simulink model "nonUsedBlocks"  (R2023b)
settings: Solver=VariableStepAuto  StartTime=0.0  StopTime=10.0  RelTol=1e-3
undefined symbols (not defined in the file or in its folder): A_bar, AEFF, B_E, C_bar, C_T, Cd_neg, Cd_pos, DiscIntNeverNeededParam, Gamma, H, L_gain, L_STROKE, M, m3PsToLpm, P_return_Pa, P_supply_Pa, PA_Pa, PB_Pa, RHO, Ts, V01, V02, W
(part 1 of 2)
settings Model: Creator=snr  LastModifiedBy=snr

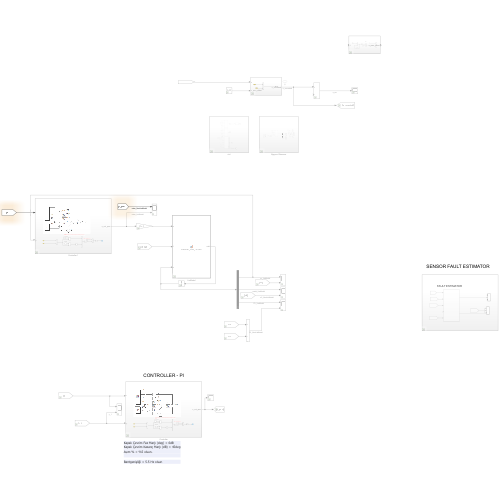
[thumbnail: Simulink's stored preview of the top-level diagram]
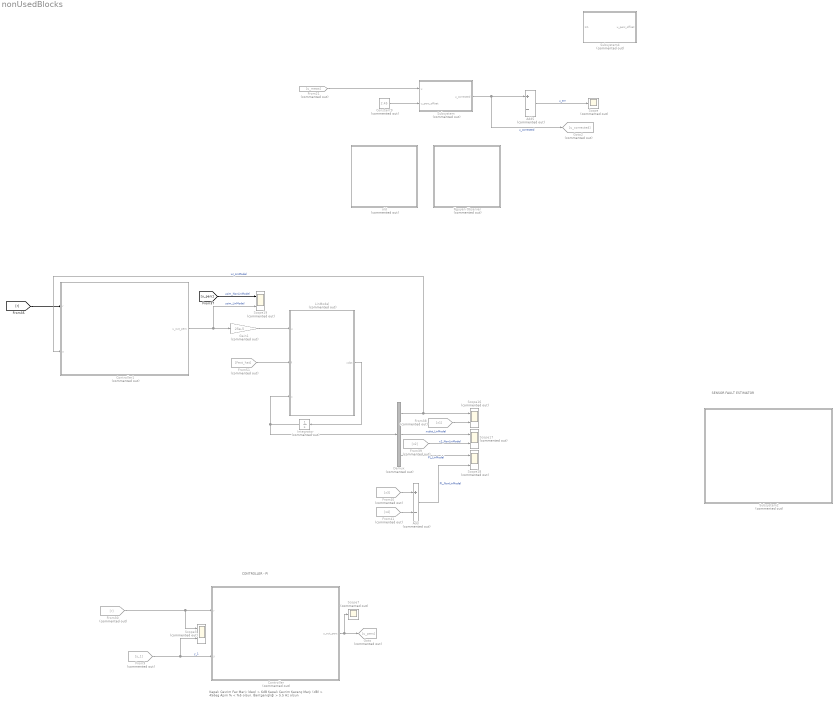
== system nonUsedBlocks ==
  note: Kapalı Çevrim Faz Marjı (deg) > 6dB
      | Kapalı Çevrim Kazanç Marjı (dB) > 45deg
      | Aşım % < %5 olsun.
      |
      | Bantgenişliği > 5.5 Hz olsun
  note: CONTROLLER - PI
  note: SENSOR FAULT ESTIMATOR
  Add : Sum  Commented=on  Inputs=+-
  Add5 : Sum  Commented=on  Inputs=+-
  Constant9 : Constant  Commented=on  Value=2.45
  Controller : Subsystem  Commented=on
  Controller1 : Subsystem  Commented=on
  Demux : Demux  Commented=on  Outputs=3
  From21 : From  Commented=on  GotoTag=u_meas
  From30 : From  Commented=on  GotoTag=r
  From38 : From  Commented=on  GotoTag=x1
  From39 : From  Commented=on  GotoTag=x2
  From40 : From  Commented=on  GotoTag=x3
  From41 : From  Commented=on  GotoTag=x4
  From51 : From  Commented=on  GotoTag=Fext_hat
  From9 : From  Commented=on  GotoTag=y_1
  Gain1 : Gain  Commented=on  Gain=25e-5
  Goto : Goto  Commented=on  GotoTag=u_perc
  Goto2 : Goto  Commented=on  GotoTag=u_corrected
  Integrator : Integrator  Commented=on  InitialCondition=[0;0;0]
  LinModel : MATLAB Function  Commented=on  TreatAsAtomicUnit=on
  Nguyen Observer : Subsystem  Commented=on
  Scope : Scope  Commented=on
  Scope{3,16..19} (5 alike) : Scope  Commented=on  NumInputPorts=2
  Scope7 : Scope  Commented=on
  Subsystem : Subsystem  Commented=on
  Subsystem2 : Subsystem  Commented=on
  Subsystem4 : Subsystem  Commented=on
  old : Subsystem  Commented=on
  wires:
  Controller1/1(u_out_perc) -> Scope19/2, Gain1/1  "usim_LinModel"
  [r] -> Controller1/1(r)
  Integrator/1 -> LinModel/3(x), Demux/1
  Demux/2 -> Scope17/1  "xcdot_LinModel"
  LinModel/1(xdot) -> Integrator/1
  From40/1 -> Add/1
  From41/1 -> Add/2
  Demux/1 -> Controller1/2(y), Scope16/1  "xc_LinModel"
  Add/1 -> Scope18/2  "PL_NonLinModel"
  Gain1/1 -> LinModel/1(u)
  From51/1 -> LinModel/2(f)
  From38/1 -> Scope16/2
  [u_perc] -> Scope19/1  "usim_NonLinModel"
  From30/1 -> Scope3/1, Controller/1(r)
  Constant9/1 -> Subsystem/2(u_perc_offset)
  Demux/3 -> Scope18/1  "PL_LinModel"
  Subsystem/1(u_corrected) -> Goto2/1, Add5/1  "u_corrected"
  Controller/1(u_out_perc) -> Scope7/1, Goto/1
  From39/1 -> Scope17/2  "x2_NonLinModel"
  Add5/1 -> Scope/1  "u_err"
  From21/1 -> Subsystem/1(u)
  From9/1 -> Scope3/2, Controller/2(y)  "y_1"

== system nonUsedBlocks/Controller ==
  note: Kontrolcü kazançları Kp : 5 - Ki :40 test düzeneğinde, Sim ortamında uygunluk için böyle ayarladım
  note: Offset - Yapmaya İhtiyaç yok
  note: Integral Gain
  note: Proportional Gain
  r : Inport  OutDataTypeStr=double
  y : Inport  Port=2  OutDataTypeStr=double
  Add : Sum
  Add1 : Sum  Inputs=+-
  Add3 : Sum
  Constant : Constant  Value=45
  Constant1 : Constant  Value=5
  Constant2 : Constant  Value=0  OutDataTypeStr=double
  Gain1 : Gain  Gain=1000
  Integrator : Integrator
  Product : Product
  Product1 : Product
  Saturation : Saturate  UpperLimit=100  LowerLimit=-100
  u_out_perc : Outport  OutDataTypeStr=double
  wires:
  Constant/1 -> Product/1
  Constant1/1 -> Product1/1
  Add1/1 -> Product1/2, Product/2  "e"
  Product/1 -> Integrator/1
  Integrator/1 -> Add/2
  r/1 -> Add1/1  "r"
  Add/1 -> Gain1/1
  y/1 -> Add1/2
  Add3/1 -> Saturation/1
  Gain1/1 -> Add3/2
  Saturation/1 -> u_out_perc/1
  Product1/1 -> Add/1
  Constant2/1 -> Add3/1

== system nonUsedBlocks/Controller1 ==
  note: Proportional Gain
  note: Integral Gain
  note: Offset - Yapmaya İhtiyaç yok
  note: Kontrolcü kazançları Kp : 5 - Ki :40 test düzeneğinde, Sim ortamında uygunluk için böyle ayarladım
  r : Inport  OutDataTypeStr=double
  y : Inport  Port=2  OutDataTypeStr=double
  Add : Sum
  Add1 : Sum  Inputs=+-
  Add3 : Sum
  Constant : Constant  Value=45
  Constant1 : Constant  Value=5
  Constant2 : Constant  Value=0  OutDataTypeStr=double
  Gain1 : Gain  Gain=1000
  Integrator : Integrator
  Product : Product
  Product1 : Product
  Saturation : Saturate  UpperLimit=100  LowerLimit=-100
  u_out_perc : Outport  OutDataTypeStr=double
  wires:
  Constant2/1 -> Add3/1
  Product1/1 -> Add/1
  Saturation/1 -> u_out_perc/1
  Gain1/1 -> Add3/2
  Add3/1 -> Saturation/1
  y/1 -> Add1/2
  Add/1 -> Gain1/1
  r/1 -> Add1/1  "r"
  Integrator/1 -> Add/2
  Product/1 -> Integrator/1
  Add1/1 -> Product/2, Product1/2  "e"
  Constant1/1 -> Product1/1
  Constant/1 -> Product/1

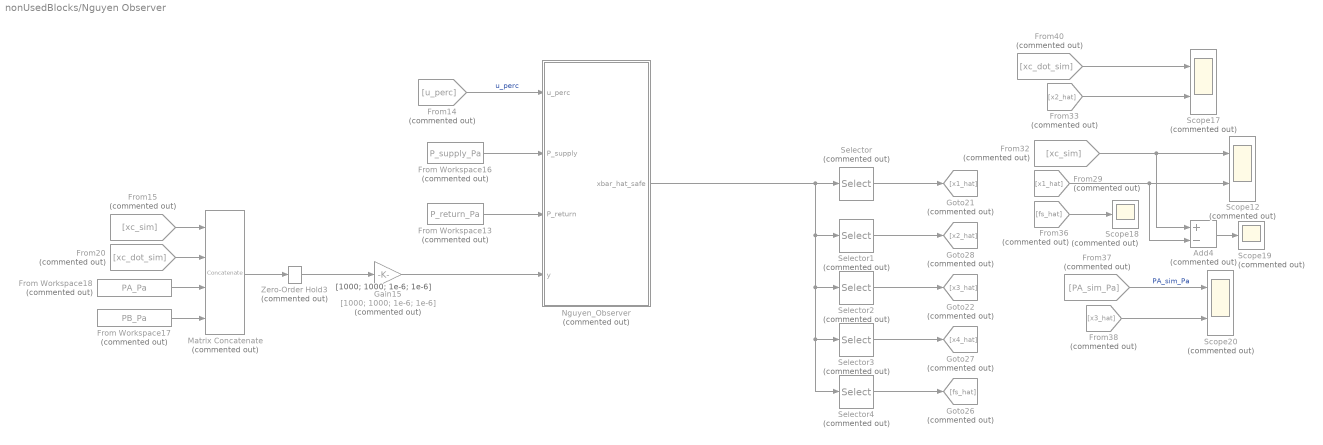
== system nonUsedBlocks/Nguyen Observer ==
  note: [1000; 1000; 1e-6; 1e-6]
  Add4 : Sum  Commented=on  Inputs=+-
  From Workspace13 : FromWorkspace  Commented=on  VariableName=P_return_Pa
  From Workspace16 : FromWorkspace  Commented=on  VariableName=P_supply_Pa
  From Workspace17 : FromWorkspace  Commented=on  VariableName=PB_Pa
  From Workspace18 : FromWorkspace  Commented=on  VariableName=PA_Pa
  From14 : From  Commented=on  GotoTag=u_perc
  From15 : From  Commented=on  GotoTag=xc_sim
  From20 : From  Commented=on  GotoTag=xc_dot_sim
  From29 : From  Commented=on  GotoTag=x1_hat
  From32 : From  Commented=on  GotoTag=xc_sim
  From33 : From  Commented=on  GotoTag=x2_hat
  From36 : From  Commented=on  GotoTag=fs_hat
  From37 : From  Commented=on  GotoTag=PA_sim_Pa
  From38 : From  Commented=on  GotoTag=x3_hat
  From40 : From  Commented=on  GotoTag=xc_dot_sim
  Gain15 : Gain  Commented=on  Gain=[1000; 1000; 1e-6; 1e-6]
  Goto21 : Goto  Commented=on  GotoTag=x1_hat
  Goto22 : Goto  Commented=on  GotoTag=x3_hat
  Goto26 : Goto  Commented=on  GotoTag=fs_hat
  Goto27 : Goto  Commented=on  GotoTag=x4_hat
  Goto28 : Goto  Commented=on  GotoTag=x2_hat
  Matrix Concatenate : Concatenate  Commented=on  NumInputs=4  Mode=Multidimensional array
  Nguyen_Observer : Subsystem  Commented=on
  Scope12 : Scope  Commented=on  NumInputPorts=2
  Scope17 : Scope  Commented=on  NumInputPorts=2
  Scope18 : Scope  Commented=on
  Scope19 : Scope  Commented=on
  Scope20 : Scope  Commented=on  NumInputPorts=2
  Selector : Selector  Commented=on  InputPortWidth=5  IndexOptions=Index vector (dialog)  Indices=1  OutputSizes=1
  Selector1 : Selector  Commented=on  InputPortWidth=5  IndexOptions=Index vector (dialog)  Indices=2  OutputSizes=1
  Selector2 : Selector  Commented=on  InputPortWidth=5  IndexOptions=Index vector (dialog)  Indices=3  OutputSizes=1
  Selector3 : Selector  Commented=on  InputPortWidth=5  IndexOptions=Index vector (dialog)  Indices=4  OutputSizes=1
  Selector4 : Selector  Commented=on  InputPortWidth=5  IndexOptions=Index vector (dialog)  Indices=5  OutputSizes=1
  Zero-Order Hold3 : ZeroOrderHold  Commented=on  SampleTime=Ts
  wires:
  From Workspace13/1 -> Nguyen_Observer/3(P_return)
  Add4/1 -> Scope19/1
  From Workspace17/1 -> Matrix Concatenate/4
  Selector4/1 -> Goto26/1
  From14/1 -> Nguyen_Observer/1(u_perc)  "u_perc"
  Selector2/1 -> Goto22/1
  Matrix Concatenate/1 -> Zero-Order Hold3/1
  From38/1 -> Scope20/2
  From Workspace16/1 -> Nguyen_Observer/2(P_supply)
  From32/1 -> Add4/1, Scope12/1
  Zero-Order Hold3/1 -> Gain15/1
  From36/1 -> Scope18/1
  From40/1 -> Scope17/1
  Gain15/1 -> Nguyen_Observer/4(y)
  From20/1 -> Matrix Concatenate/2
  From15/1 -> Matrix Concatenate/1
  Selector/1 -> Goto21/1
  Selector3/1 -> Goto27/1
  From37/1 -> Scope20/1  "PA_sim_Pa"
  Selector1/1 -> Goto28/1
  From Workspace18/1 -> Matrix Concatenate/3
  Nguyen_Observer/1(xbar_hat_safe) -> Selector4/1, Selector3/1, Selector2/1, Selector1/1, Selector/1
  From33/1 -> Scope17/2
  From29/1 -> Add4/2, Scope12/2

== system nonUsedBlocks/Subsystem ==
  u : Inport  OutDataTypeStr=double
  u_perc_offset : Inport  Port=2  OutDataTypeStr=double
  Add : Sum  Inputs=+-
  u_corrected : Outport
  wires:
  u/1 -> Add/1
  u_perc_offset/1 -> Add/2
  Add/1 -> u_corrected/1

== system nonUsedBlocks/Subsystem2 ==
  note: FAULT ESTIMATOR
  From14 : From  Commented=on  GotoTag=u_perc
  From15 : From  Commented=on  GotoTag=PA_sim_Pa
  From20 : From  Commented=on  GotoTag=PB_sim_Pa
  From29 : From  Commented=on  GotoTag=fs_real
  From33 : From  Commented=on  GotoTag=xc_dot_sim
  Scope12 : Scope  Commented=on  NumInputPorts=3
  Scope17 : Scope  Commented=on  NumInputPorts=3
  Subsystem3 : Subsystem  Commented=on
  wires:
  Subsystem3/2(Out1) -> Scope17/1
  From20/1 -> Subsystem3/3(PB_Pa)  "PB_sim_Pa"
  From29/1 -> Subsystem3/5(fs_real)
  From14/1 -> Subsystem3/1(u_real)  "u_perc"
  From33/1 -> Scope17/2
  From15/1 -> Subsystem3/2(PA_Pa)
  Subsystem3/1(x_bar) -> Scope12/2  "x_bar"

== system nonUsedBlocks/Subsystem4 ==
  In1 : Inport
  Add : Sum
  Constant : Constant
  Constant1 : Constant  Value=100
  Relational Operator : RelationalOperator  OutDataTypeStr=boolean  RndMeth=Simplest  InputSameDT=off
  Saturation : Saturate  UpperLimit=100  LowerLimit=0
  Switch : Switch  Criteria=u2 ~= 0  SaturateOnIntegerOverflow=off  InputSameDT=off
  Unit Delay : UnitDelay  SampleTime=-1  HasFrameUpgradeWarning=on
  u_perc_offset : Outport
  wires:
  Constant/1 -> Add/1
  Add/1 -> Unit Delay/1, Saturation/1
  Unit Delay/1 -> Add/2
  Saturation/1 -> Relational Operator/1
  Constant1/1 -> Relational Operator/2
  Relational Operator/1 -> Switch/2
  In1/1 -> Switch/1

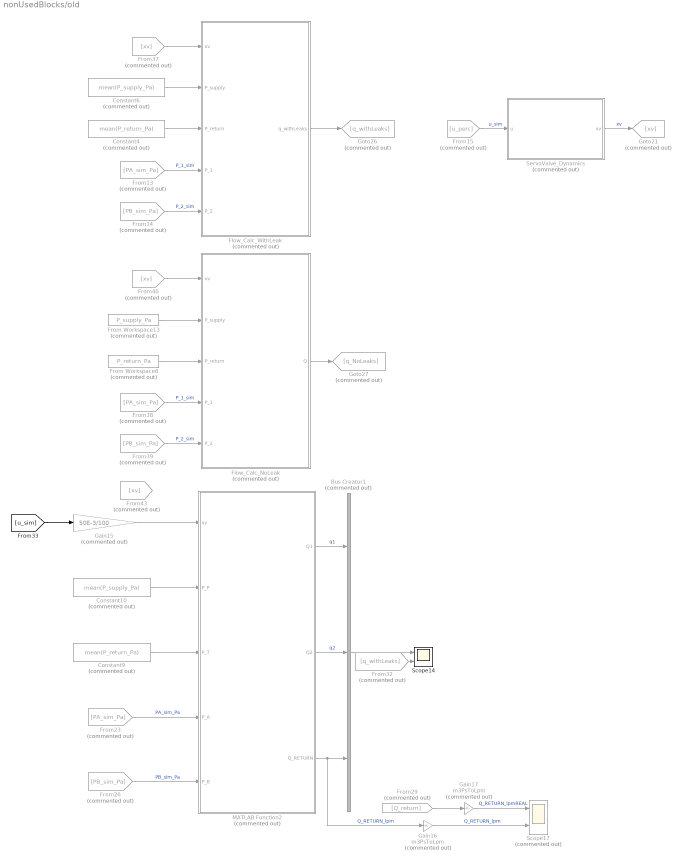
== system nonUsedBlocks/old ==
  Bus Creator1 : BusCreator  Commented=on  Inputs=3
  Constant10 : Constant  Commented=on  Value=mean(P_supply_Pa)
  Constant4 : Constant  Commented=on  Value=mean(P_return_Pa)
  Constant6 : Constant  Commented=on  Value=mean(P_supply_Pa)
  Constant9 : Constant  Commented=on  Value=mean(P_return_Pa)
  Flow_Calc_NoLeak : Subsystem  Commented=on
  Flow_Calc_WithLeak : Subsystem  Commented=on
  From Workspace13 : FromWorkspace  Commented=on  VariableName=P_supply_Pa
  From Workspace8 : FromWorkspace  Commented=on  VariableName=P_return_Pa
  From13 : From  Commented=on  GotoTag=PA_sim_Pa
  From14 : From  Commented=on  GotoTag=PB_sim_Pa
  From15 : From  Commented=on  GotoTag=u_perc
  From23 : From  Commented=on  GotoTag=PA_sim_Pa
  From26 : From  Commented=on  GotoTag=PB_sim_Pa
  From29 : From  Commented=on  GotoTag=Q_return
  From32 : From  Commented=on  GotoTag=q_withLeaks
  From37 : From  Commented=on  GotoTag=xv
  From38 : From  Commented=on  GotoTag=PA_sim_Pa
  From39 : From  Commented=on  GotoTag=PB_sim_Pa
  From40 : From  Commented=on  GotoTag=xv
  From43 : From  Commented=on  GotoTag=xv
  Gain15 : Gain  Commented=on  Gain=50E-3/100
  Gain16 : Gain  Commented=on  Gain=m3PsToLpm
  Gain17 : Gain  Commented=on  Gain=m3PsToLpm
  Goto21 : Goto  Commented=on  GotoTag=xv
  Goto26 : Goto  Commented=on  GotoTag=q_withLeaks
  Goto27 : Goto  Commented=on  GotoTag=q_NoLeaks
  MATLAB Function2 : MATLAB Function  Commented=on  TreatAsAtomicUnit=on
  Scope14 : Scope  NumInputPorts=2
  Scope17 : Scope  Commented=on  NumInputPorts=2
  ServoValve_Dynamics : Subsystem  Commented=on
  wires:
  Constant9/1 -> MATLAB Function2/3(P_T)
  From32/1 -> Scope14/2
  Constant4/1 -> Flow_Calc_WithLeak/3(P_return)
  From26/1 -> MATLAB Function2/5(P_B)  "PB_sim_Pa"
  From Workspace13/1 -> Flow_Calc_NoLeak/2(P_supply)
  From29/1 -> Gain17/1
  Gain15/1 -> MATLAB Function2/1(xv)
  Bus Creator1/1 -> Scope14/1
  From37/1 -> Flow_Calc_WithLeak/1(xv)
  Constant10/1 -> MATLAB Function2/2(P_P)
  From Workspace8/1 -> Flow_Calc_NoLeak/3(P_return)
  MATLAB Function2/3(Q_RETURN) -> Gain16/1, Bus Creator1/3  "Q_RETURN_lpm"
  From23/1 -> MATLAB Function2/4(P_A)  "PA_sim_Pa"
  Gain16/1 -> Scope17/2  "Q_RETURN_lpm"
  MATLAB Function2/1(Q1) -> Bus Creator1/1  "q1"
  MATLAB Function2/2(Q2) -> Bus Creator1/2  "q2"
  From14/1 -> Flow_Calc_WithLeak/5(P_2)  "P_2_sim"
  From39/1 -> Flow_Calc_NoLeak/5(P_2)  "P_2_sim"
  Flow_Calc_NoLeak/1(Q) -> Goto27/1
  Flow_Calc_WithLeak/1(q_withLeaks) -> Goto26/1
  From40/1 -> Flow_Calc_NoLeak/1(xv)
  [u_sim] -> Gain15/1
  Constant6/1 -> Flow_Calc_WithLeak/2(P_supply)
  From38/1 -> Flow_Calc_NoLeak/4(P_1)  "P_1_sim"
  From13/1 -> Flow_Calc_WithLeak/4(P_1)  "P_1_sim"
  Gain17/1 -> Scope17/1  "Q_RETURN_lpmREAL"
  ServoValve_Dynamics/1(xv) -> Goto21/1  "xv"
  From15/1 -> ServoValve_Dynamics/1(u)  "u_sim"

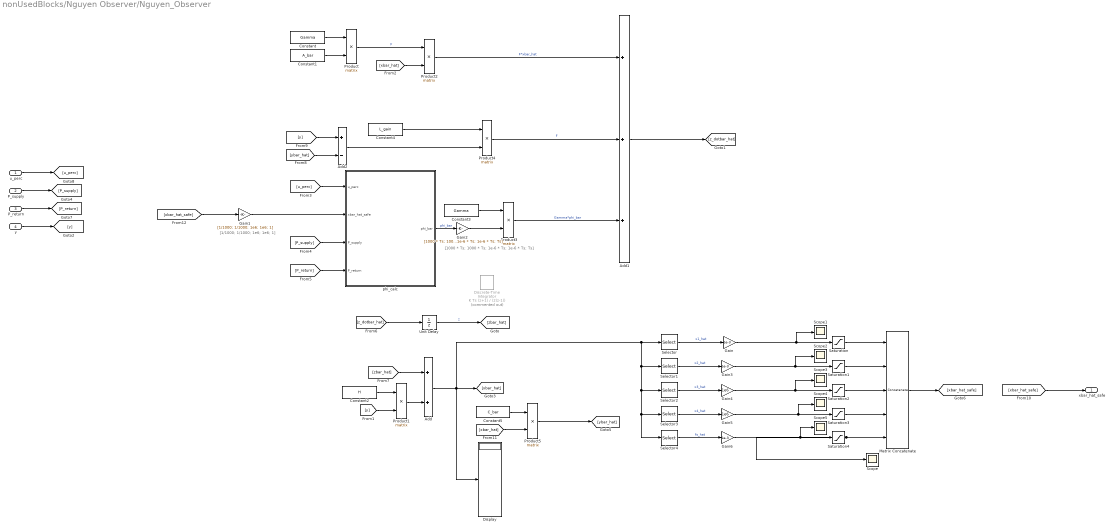
== system nonUsedBlocks/Nguyen Observer/Nguyen_Observer ==
  note: [1000 * Ts; 1000 * Ts; 1e-6 * Ts; 1e-6 * Ts; Ts]
  note: [1/1000; 1/1000; 1e6; 1e6; 1]
  u_perc : Inport  PortDimensions=[1,1]
  P_supply : Inport  Port=2  OutDataTypeStr=double
  P_return : Inport  Port=3  OutDataTypeStr=double
  y : Inport  Port=4  PortDimensions=[4,1]
  Add : Sum
  Add1 : Sum  Inputs=+++
  Add2 : Sum  Inputs=+-
  Constant : Constant  Value=Gamma
  Constant1 : Constant  Value=A_bar
  Constant2 : Constant  Value=H
  Constant3 : Constant  Value=Gamma
  Constant4 : Constant  Value=L_gain
  Constant5 : Constant  Value=C_bar
  Discrete-Time Integrator : DiscreteIntegrator  Commented=on  IntegratorMethod=Integration: Trapezoidal  InitialCondition=[0,0,PA_Pa.Data(1)*1e-6,PB_Pa.Data(1)*1e-6,0]'  SampleTime=-1  ICPrevOutput=DiscIntNeverNeededParam  ICPrevScaledInput=DiscIntNeverNeededParam
  Display : Display
  Gain : Gain  Gain=1e-3
  Gain1 : Gain  Gain=[1/1000; 1/1000; 1e6; 1e6; 1]
  Gain2 : Gain  Gain=[1000 * Ts; 1000 * Ts; 1e-6 * Ts; 1e-6 * Ts; Ts]
  Gain3 : Gain  Gain=1e-3
  Gain4 : Gain  Gain=1e6
  Gain5 : Gain  Gain=1e6
  Gain6 : Gain  Gain=1e-3
  Matrix Concatenate : Concatenate  NumInputs=5  Mode=Multidimensional array
  Product{,1..5} (6 alike) : Product  Multiplication=Matrix(*)
  Saturation : Saturate  UpperLimit=L_STROKE  LowerLimit=-L_STROKE
  Saturation1 : Saturate  UpperLimit=2  LowerLimit=-2
  Saturation2 : Saturate  UpperLimit=200e5  LowerLimit=4e5
  Saturation3 : Saturate  UpperLimit=200e5  LowerLimit=4e5
  Saturation4 : Saturate  UpperLimit=L_STROKE  LowerLimit=-L_STROKE
  Scope{,1..5} (6 alike) : Scope
  Selector : Selector  InputPortWidth=5  IndexOptions=Index vector (dialog)  Indices=1  OutputSizes=1
  Selector1 : Selector  InputPortWidth=5  IndexOptions=Index vector (dialog)  Indices=2  OutputSizes=1
  Selector2 : Selector  InputPortWidth=5  IndexOptions=Index vector (dialog)  Indices=3  OutputSizes=1
  Selector3 : Selector  InputPortWidth=5  IndexOptions=Index vector (dialog)  Indices=4  OutputSizes=1
  Selector4 : Selector  InputPortWidth=5  IndexOptions=Index vector (dialog)  Indices=5  OutputSizes=1
  Unit Delay : UnitDelay  InitialCondition=[0,0,PA_Pa.Data(1)*1e-6,PB_Pa.Data(1)*1e-6,0]'  SampleTime=Ts  HasFrameUpgradeWarning=on
  phi_calc : Subsystem
  xbar_hat_safe : Outport
  wires:
  [y] -> Add2/1
  Product3/1 -> Add1/3  "Gamma*phi_bar"
  [u_perc] -> phi_calc/1(u_perc)
  Add2/1 -> Product4/2
  u_perc/1 -> [u_perc]
  Constant3/1 -> Product3/1
  Unit Delay/1 -> [zbar_hat]  "z"
  [ybar_hat] -> Add2/2
  Constant2/1 -> Product1/1
  Product/1 -> Product2/1  "F"
  [P_return] -> phi_calc/4(P_return)
  Constant1/1 -> Product/2
  Product2/1 -> Add1/1  "F*xbar_hat"
  Constant/1 -> Product/1
  [xbar_hat] -> Product2/2
  P_return/1 -> [P_return]
  [y] -> Product1/2
  [zbar_hat] -> Add/1
  y/1 -> [y]
  Add1/1 -> [z_dotbar_hat]
  Product4/1 -> Add1/2  "F"
  Product1/1 -> Add/2
  P_supply/1 -> [P_supply]
  phi_calc/1(phi_bar) -> Gain2/1  "phi_bar"
  [P_supply] -> phi_calc/3(P_supply)
  [z_dotbar_hat] -> Unit Delay/1
  [xbar_hat_safe] -> xbar_hat_safe/1
  Constant5/1 -> Product5/1
  [xbar_hat] -> Product5/2
  Product5/1 -> [ybar_hat]
  Selector3/1 -> Gain5/1  "x4_hat"
  Selector2/1 -> Gain4/1  "x3_hat"
  Selector1/1 -> Gain3/1  "x2_hat"
  Saturation/1 -> Matrix Concatenate/1
  Saturation1/1 -> Matrix Concatenate/2
  Saturation2/1 -> Matrix Concatenate/3
  Saturation3/1 -> Matrix Concatenate/4
  Saturation4/1 -> Scope/1, Matrix Concatenate/5
  Matrix Concatenate/1 -> [xbar_hat_safe]
  Selector4/1 -> Gain6/1  "fs_hat"
  Selector/1 -> Gain/1  "x1_hat"
  Constant4/1 -> Product4/1
  Add/1 -> Selector3/1, Selector4/1, Selector2/1, Selector1/1, Selector/1, [xbar_hat], Display/1
  [xbar_hat_safe] -> Gain1/1
  Gain1/1 -> phi_calc/2(xbar_hat_safe)
  Gain2/1 -> Product3/2
  Gain/1 -> Scope1/1, Saturation/1
  Gain3/1 -> Scope2/1, Saturation1/1
  Gain4/1 -> Saturation2/1, Scope3/1
  Gain5/1 -> Saturation3/1, Scope4/1
  Gain6/1 -> Scope5/1, Saturation4/1

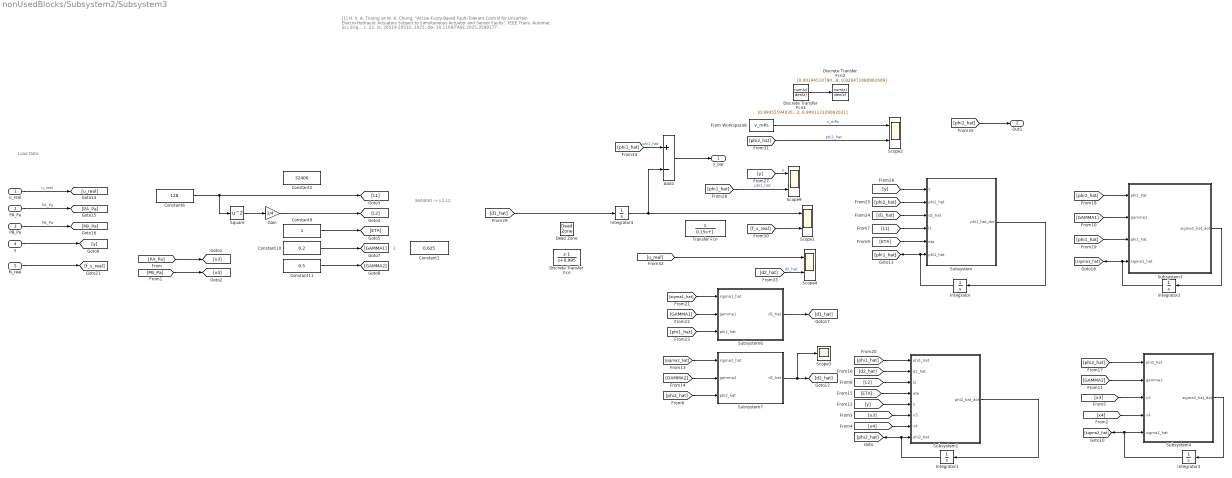
== system nonUsedBlocks/Subsystem2/Subsystem3 ==
  note: [1]
      | H. V. A. Truong ve W. K. Chung, “Active Fuzzy-Based Fault-Tolerant Control for Uncertain Electro-Hydraulic Actuators Subject to Simultaneous Actuator and Sensor Faults”, IEEE Trans. Automat. Sci. Eng. , c. 22, ss. 20519-20532, 2025, doi: 10.1109/TASE.2025.3599177 .
  note: 2
  note: 360/850 -> L1,L2
  note: Load Data
  u_real : Inport
  PA_Pa : Inport  Port=2
  PB_Pa : Inport  Port=3
  y : Inport  Port=4
  fs_real : Inport  Port=5
  Add1 : Sum  Inputs=+-
  Constant1 : Constant  Value=0.625
  Constant10 : Constant  Value=0.2
  Constant11 : Constant  Value=0.5
  Constant2 : Constant  Value=32400
  Constant6 : Constant  Value=128
  Constant9 : Constant
  Dead Zone : DeadZone  LowerValue=-0.01  UpperValue=0.01
  Discrete Transfer Fcn : DiscreteTransferFcn  Numerator=[1 -1]  Denominator=[1 0.995]
  Discrete Transfer Fcn1 : DiscreteTransferFcn  Numerator=[0.999555940307616, -1.999111880615232, 0.999555940307616]  Denominator=[1.000000000000000, -1.999111432168433, 0.999112329062031]
  Discrete Transfer Fcn2 : DiscreteTransferFcn  Numerator=[0.001945107908955, 0.003890215817911, 0.001945107908955]  Denominator=[1.000000000000000, -1.812690649346788, 0.820471080982609]
  From Workspace6 : FromWorkspace  VariableName=v_mPs
  Gain : Gain  Gain=1/4
  Integrator{,1..4} (5 alike) : Integrator
  Scope{1..2,4,9} (4 alike) : Scope  NumInputPorts=2
  Scope3 : Scope
  Square : Math  Operator=square
  Subsystem : Subsystem
  Subsystem1 : Subsystem
  Subsystem3 : Subsystem
  Subsystem4 : Subsystem
  Subsystem6 : Subsystem
  Subsystem7 : Subsystem
  Transfer Fcn : TransferFcn  Denominator=[0.15 1]
  x_bar : Outport
  Out1 : Outport  Port=2
  wires:
  [u_real] -> Scope4/1
  Subsystem4/1(sigma2_hat_dot) -> Integrator3/1
  Constant6/1 -> Square/1, [L1]
  [y] -> Subsystem/1(y)
  Constant9/1 -> [ETA]
  [GAMMA2] -> Subsystem7/2(gamma2)
  [GAMMA1] -> Subsystem3/2(gamma1)
  Subsystem/1(phi1_hat_dot) -> Integrator/1
  Gain/1 -> [L2]
  [GAMMA1] -> Subsystem6/2(gamma1)
  [y] -> Subsystem1/5(y)
  Constant10/1 -> [GAMMA1]
  y/1 -> [y]
  [GAMMA2] -> Subsystem4/2(gamma2)
  Subsystem7/1(d2_hat) -> Scope3/1, [d2_hat]
  [L2] -> Subsystem1/3(l2)
  Subsystem6/1(d1_hat) -> [d1_hat]
  [phi1_hat] -> Subsystem3/3(phi1_hat)
  [ETA] -> Subsystem/5(eta)
  [phi1_hat] -> Scope9/2  "phi1_hat"
  Integrator/1 -> [phi1_hat], Subsystem/6(phi1_hat)
  [d2_hat] -> Subsystem1/2(d2_hat)
  Constant11/1 -> [GAMMA2]
  [d2_hat] -> Scope4/2  "d2_hat"
  [phi2_hat] -> Subsystem7/3(phi2_hat)
  [y] -> Scope9/1  "y"
  [phi2_hat] -> Subsystem4/1(phi2_hat)
  [sigma1_hat] -> Subsystem6/1(sigma1_hat)
  [L1] -> Subsystem/4(l1)
  Integrator2/1 -> [sigma1_hat], Subsystem3/4(sigma1_hat)
  [PA_Pa] -> [x3]
  [x3] -> Subsystem1/6(x3)
  PB_Pa/1 -> [PB_Pa]  "PB_Pa"
  u_real/1 -> [u_real]  "u_real"
  Subsystem3/1(sigma1_hat_dot) -> Integrator2/1
  [ETA] -> Subsystem1/4(eta)
  [phi1_hat] -> Subsystem6/3(phi1_hat)
  Integrator3/1 -> Subsystem4/5(sigma2_hat), [sigma2_hat]
  [sigma2_hat] -> Subsystem7/1(sigma2_hat)
  [x3] -> Subsystem4/3(x3)
  [x4] -> Subsystem4/4(x4)
  [d1_hat] -> Subsystem/3(d1_hat)
  From Workspace6/1 -> Scope2/1  "v_mPs"
  [phi1_hat] -> Subsystem1/1(phi1_hat)
  [phi2_hat] -> Subsystem/2(phi2_hat)
  [phi2_hat] -> Subsystem3/1(phi2_hat)
  [x4] -> Subsystem1/7(x4)
  PA_Pa/1 -> [PA_Pa]  "PA_Pa"
  [PB_Pa] -> [x4]
  [phi1_hat] -> Add1/1  "phi1_hat"
  Add1/1 -> x_bar/1
  fs_real/1 -> [f_s_real]
  [phi2_hat] -> Out1/1
  Subsystem1/1(phi2_hat_dot) -> Integrator1/1
  Integrator1/1 -> Subsystem1/8(phi2_hat), [phi2_hat]
  Square/1 -> Gain/1
  [d1_hat] -> Integrator4/1
  Integrator4/1 -> Scope1/1, Add1/2
  [f_s_real] -> Scope1/2
  Discrete Transfer Fcn1/1 -> Discrete Transfer Fcn2/1
  [phi2_hat] -> Scope2/2  "phi2_hat"

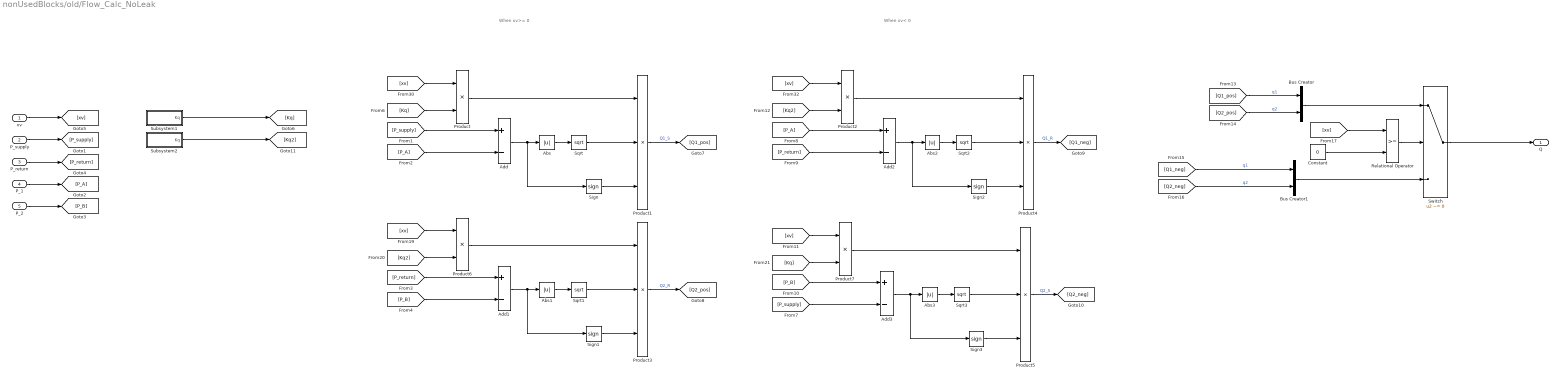
== system nonUsedBlocks/old/Flow_Calc_NoLeak ==
  note: When xv< 0
  note: When xv>= 0
  xv : Inport  OutDataTypeStr=double
  P_supply : Inport  Port=2  OutDataTypeStr=double
  P_return : Inport  Port=3  OutDataTypeStr=double
  P_1 : Inport  Port=4  OutDataTypeStr=double
  P_2 : Inport  Port=5  OutDataTypeStr=double
  Abs{,1..3} (4 alike) : Abs  SaturateOnIntegerOverflow=off
  Add{,1..3} (4 alike) : Sum  Inputs=+-
  Bus Creator : BusCreator  Inputs=2
  Bus Creator1 : BusCreator  Inputs=2
  Constant : Constant  Value=0  OutDataTypeStr=double
  Product{,2,6..7} (4 alike) : Product
  Product{1,3..5} (4 alike) : Product  Inputs=3
  Relational Operator : RelationalOperator  OutDataTypeStr=boolean  RndMeth=Simplest  InputSameDT=off
  Sign{,1..3} (4 alike) : Signum
  Sqrt{,1..3} (4 alike) : Sqrt
  Subsystem1 : Subsystem
  Subsystem2 : Subsystem
  Switch : Switch  Criteria=u2 ~= 0  SaturateOnIntegerOverflow=off  InputSameDT=off
  Q : Outport  OutDataTypeStr=double
  wires:
  Subsystem2/1(Kq) -> [Kq2]
  Subsystem1/1(Kq) -> [Kq]
  Product5/1 -> [Q2_neg]  "Q2_S"
  Product4/1 -> [Q1_neg]  "Q1_R"
  Product3/1 -> [Q2_pos]  "Q2_R"
  Product1/1 -> [Q1_pos]  "Q1_S"
  Switch/1 -> Q/1
  [xv] -> Product/1
  [Q1_neg] -> Bus Creator1/1  "q1"
  [Q2_pos] -> Bus Creator/2  "q2"
  Product7/1 -> Product5/1
  [xv] -> Product7/1
  [Kq] -> Product7/2
  Product6/1 -> Product3/1
  [Kq2] -> Product6/2
  [xv] -> Product6/1
  Bus Creator1/1 -> Switch/3
  Bus Creator/1 -> Switch/1
  Relational Operator/1 -> Switch/2
  Constant/1 -> Relational Operator/2
  [xv] -> Relational Operator/1
  [Q2_neg] -> Bus Creator1/2  "q2"
  [Q1_pos] -> Bus Creator/1  "q1"
  [P_supply] -> Add3/2
  [P_B] -> Add3/1
  [P_return] -> Add2/2
  [P_A] -> Add2/1
  Product2/1 -> Product4/1
  Sqrt2/1 -> Product4/2
  Abs2/1 -> Sqrt2/1
  Add2/1 -> Abs2/1, Sign2/1
  Sign2/1 -> Product4/3
  Sign3/1 -> Product5/3
  Add3/1 -> Sign3/1, Abs3/1
  Abs3/1 -> Sqrt3/1
  Sqrt3/1 -> Product5/2
  [Kq2] -> Product2/2
  [xv] -> Product2/1
  xv/1 -> [xv]
  P_return/1 -> [P_return]
  P_2/1 -> [P_B]
  P_1/1 -> [P_A]
  P_supply/1 -> [P_supply]
  [P_B] -> Add1/2
  [P_return] -> Add1/1
  [Kq] -> Product/2
  Sqrt1/1 -> Product3/2
  Abs1/1 -> Sqrt1/1
  Add1/1 -> Abs1/1, Sign1/1
  Sign1/1 -> Product3/3
  Sign/1 -> Product1/3
  Add/1 -> Sign/1, Abs/1
  Abs/1 -> Sqrt/1
  Sqrt/1 -> Product1/2
  Product/1 -> Product1/1
  [P_A] -> Add/2
  [P_supply] -> Add/1

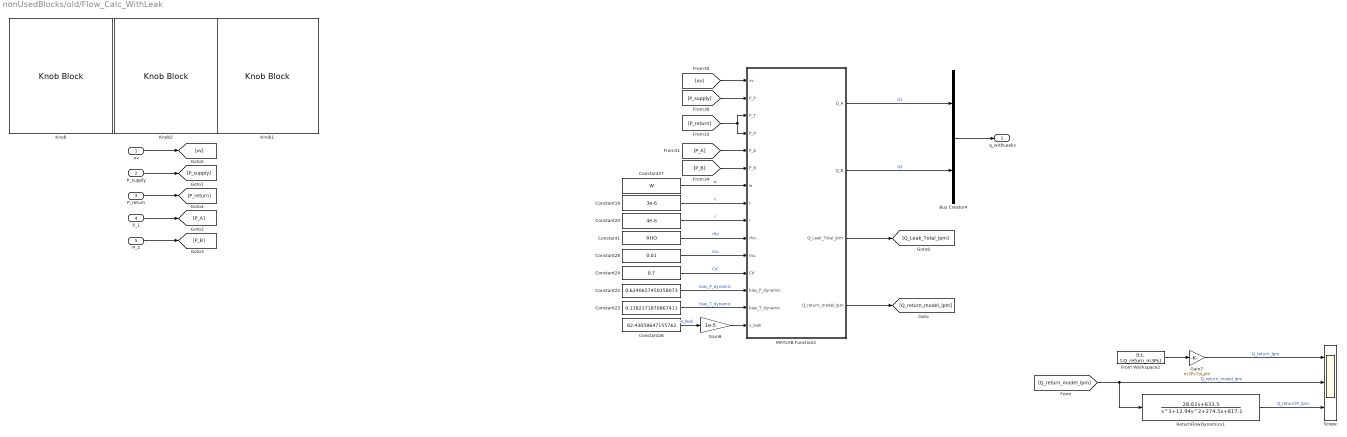
== system nonUsedBlocks/old/Flow_Calc_WithLeak ==
  xv : Inport  OutDataTypeStr=double
  P_supply : Inport  Port=2  OutDataTypeStr=double
  P_return : Inport  Port=3  OutDataTypeStr=double
  P_1 : Inport  Port=4  OutDataTypeStr=double
  P_2 : Inport  Port=5  OutDataTypeStr=double
  Bus Creator4 : BusCreator  Inputs=2
  Constant1 : Constant  Value=RHO
  Constant19 : Constant  Value=3e-6
  Constant20 : Constant  Value=4e-6
  Constant22 : Constant  Value=0.6240657450358073
  Constant23 : Constant  Value=0.1382171870867411
  Constant24 : Constant  Value=0.7
  Constant26 : Constant  Value=82.43058647155762
  Constant27 : Constant  Value=W
  Constant28 : Constant  Value=0.01
  From Workspace2 : FromWorkspace  VariableName=[t.t, t.Q_return_m3Ps]
  Gain7 : Gain  Gain=m3PsToLpm
  Gain8 : Gain  Gain=1e-5
  Knob : KnobBlock  ScaleMin=0.1  ScaleMax=2
  Knob1 : KnobBlock  ScaleMin=0.1
  Knob2 : KnobBlock  ScaleMin=0.1  ScaleMax=2
  MATLAB Function2 : MATLAB Function  TreatAsAtomicUnit=on
  ReturnFlowDynamics1 : TransferFcn  Numerator=[28.61 633.5]  Denominator=[1 12.94 274.5 817.1]
  Scope : Scope  NumInputPorts=3
  q_withLeaks : Outport  OutDataTypeStr=double
  wires:
  P_supply/1 -> [P_supply]
  P_1/1 -> [P_A]
  P_2/1 -> [P_B]
  P_return/1 -> [P_return]
  xv/1 -> [xv]
  [xv] -> MATLAB Function2/1(xv)
  [P_supply] -> MATLAB Function2/2(P_P)
  [P_return] -> MATLAB Function2/3(P_T), MATLAB Function2/4(P_R)
  [P_A] -> MATLAB Function2/5(P_A)
  [P_B] -> MATLAB Function2/6(P_B)
  Constant27/1 -> MATLAB Function2/7(w)  "w"
  Constant19/1 -> MATLAB Function2/8(c)  "c"
  Constant20/1 -> MATLAB Function2/9(r)  "r"
  Constant1/1 -> MATLAB Function2/10(rho)  "rho"
  Constant28/1 -> MATLAB Function2/11(mu)  "mu"
  Constant24/1 -> MATLAB Function2/12(Cd)  "Cd"
  Constant22/1 -> MATLAB Function2/13(bias_P_dynamic)  "bias_P_dynamic"
  Constant23/1 -> MATLAB Function2/14(bias_T_dynamic)  "bias_T_dynamic"
  From Workspace2/1 -> Gain7/1
  Bus Creator4/1 -> q_withLeaks/1
  MATLAB Function2/1(Q_A) -> Bus Creator4/1  "q1"
  MATLAB Function2/2(Q_B) -> Bus Creator4/2  "q2"
  Constant26/1 -> Gain8/1  "x_leak"
  Gain8/1 -> MATLAB Function2/15(x_leak)
  MATLAB Function2/4(Q_return_model_lpm) -> [Q_return_model_lpm]
  MATLAB Function2/3(Q_Leak_Total_lpm) -> [Q_Leak_Total_lpm]
  Gain7/1 -> Scope/1  "Q_return_lpm"
  ReturnFlowDynamics1/1 -> Scope/3  "Q_returnTF_lpm"
  [Q_return_model_lpm] -> ReturnFlowDynamics1/1, Scope/2  "Q_return_model_lpm"

== system nonUsedBlocks/old/ServoValve_Dynamics ==
  note: Deadband
  u : Inport  OutDataTypeStr=double
  Convert_SpoolPosition : Subsystem
  Dead Zone : DeadZone  LowerValue=-0.05  UpperValue=0.05
  Subsystem : Subsystem  Commented=on
  Valve Dynamics : TransferFcn  Numerator=[2.0884e+06]  Denominator=[1 2*1*1.4451e+03 2.0884e+06]
  xv : Outport  OutDataTypeStr=double
  wires:
  Dead Zone/1 -> Valve Dynamics/1
  u/1 -> Dead Zone/1
  Convert_SpoolPosition/1(xv) -> xv/1
  Valve Dynamics/1 -> Convert_SpoolPosition/1(u_perc)

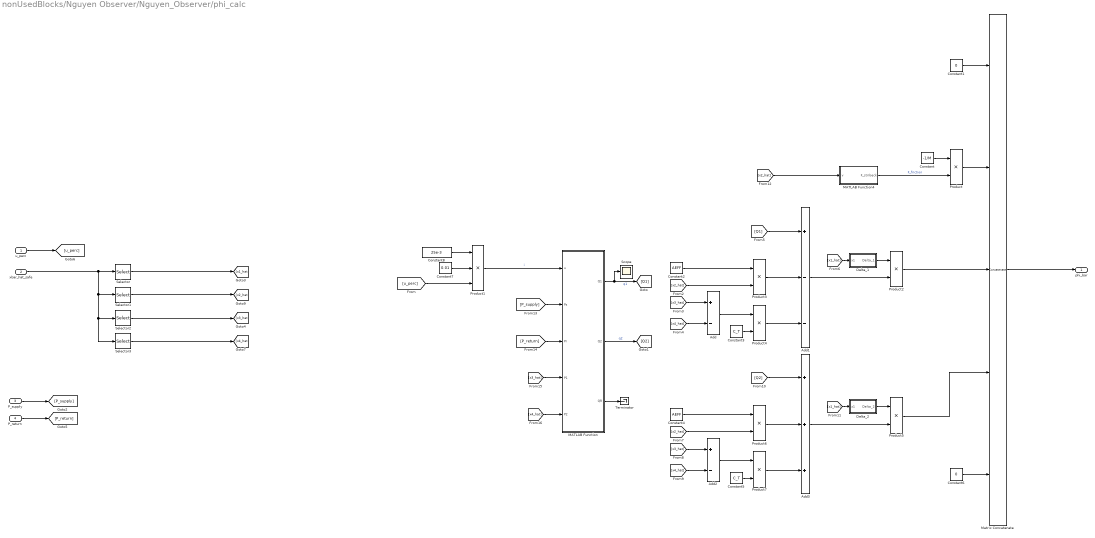
== system nonUsedBlocks/Nguyen Observer/Nguyen_Observer/phi_calc ==
  u_perc : Inport
  xbar_hat_safe : Inport  Port=2
  P_supply : Inport  Port=3  OutDataTypeStr=double
  P_return : Inport  Port=4  OutDataTypeStr=double
  Add : Sum  Inputs=+-
  Add1 : Sum  Inputs=+--
  Add2 : Sum  Inputs=+-
  Add3 : Sum  Inputs=+++
  Constant : Constant  Value=-1/M
  Constant1 : Constant  Value=0
  Constant2 : Constant  Value=AEFF
  Constant3 : Constant  Value=C_T
  Constant4 : Constant  Value=AEFF
  Constant5 : Constant  Value=C_T
  Constant6 : Constant  Value=0
  Constant7 : Constant  Value=0.01
  Constant8 : Constant  Value=25e-3
  Delta_1 : Subsystem
  Delta_2 : Subsystem
  MATLAB Function : MATLAB Function  TreatAsAtomicUnit=on
  MATLAB Function4 : MATLAB Function  TreatAsAtomicUnit=on
  Matrix Concatenate : Concatenate  NumInputs=5  Mode=Multidimensional array
  Product{,2..7} (7 alike) : Product
  Product1 : Product  Inputs=3
  Scope : Scope
  Selector : Selector  InputPortWidth=5  IndexOptions=Index vector (dialog)  Indices=1  OutputSizes=1
  Selector1 : Selector  InputPortWidth=5  IndexOptions=Index vector (dialog)  Indices=2  OutputSizes=1
  Selector2 : Selector  InputPortWidth=5  IndexOptions=Index vector (dialog)  Indices=3  OutputSizes=1
  Selector3 : Selector  InputPortWidth=5  IndexOptions=Index vector (dialog)  Indices=4  OutputSizes=1
  Terminator : Terminator
  phi_bar : Outport
  wires:
  MATLAB Function4/1(F_stribeck) -> Product/2  "F_friction"
  Constant/1 -> Product/1
  MATLAB Function/1(Q1) -> Scope/1, [Q1]  "q1"
  MATLAB Function/2(Q2) -> [Q2]  "q2"
  [Q1] -> Add1/1
  [x2_hat] -> Product3/2
  [x4_hat] -> Add/2
  [x3_hat] -> Add/1
  Add/1 -> Product4/1
  Constant3/1 -> Product4/2
  Product3/1 -> Add1/2
  Product4/1 -> Add1/3
  Add1/1 -> Product2/2
  Delta_1/1(Delta_1) -> Product2/1
  [x1_hat] -> Delta_1/1(x1)
  [x1_hat] -> Delta_2/1(x1)
  Delta_2/1(Delta_2) -> Product5/1
  Add3/1 -> Product5/2
  Product7/1 -> Add3/3
  Product6/1 -> Add3/2
  Constant5/1 -> Product7/2
  Add2/1 -> Product7/1
  [x3_hat] -> Add2/1
  [x4_hat] -> Add2/2
  [x2_hat] -> Product6/2
  [Q2] -> Add3/1
  Constant6/1 -> Matrix Concatenate/5
  Product5/1 -> Matrix Concatenate/4
  Product/1 -> Matrix Concatenate/2
  Constant1/1 -> Matrix Concatenate/1
  Constant7/1 -> Product1/2
  Constant8/1 -> Product1/1
  Product1/1 -> MATLAB Function/1(u)  "i"
  u_perc/1 -> [u_perc]
  P_return/1 -> [P_return]
  P_supply/1 -> [P_supply]
  [u_perc] -> Product1/3
  [P_supply] -> MATLAB Function/2(Ps)
  [P_return] -> MATLAB Function/3(Pr)
  [x3_hat] -> MATLAB Function/4(P1)
  [x4_hat] -> MATLAB Function/5(P2)
  MATLAB Function/3(QR) -> Terminator/1
  Matrix Concatenate/1 -> phi_bar/1
  Selector/1 -> [x1_hat]
  Selector1/1 -> [x2_hat]
  Selector2/1 -> [x3_hat]
  Selector3/1 -> [x4_hat]
  Constant2/1 -> Product3/1
  Constant4/1 -> Product6/1
  Product2/1 -> Matrix Concatenate/3
  [x2_hat] -> MATLAB Function4/1(v)
  xbar_hat_safe/1 -> Selector3/1, Selector2/1, Selector1/1, Selector/1

== system nonUsedBlocks/Subsystem2/Subsystem3/Subsystem ==
  y : Inport
  phi2_hat : Inport  Port=2
  d1_hat : Inport  Port=3
  l1 : Inport  Port=4
  eta : Inport  Port=5
  phi1_hat : Inport  Port=6
  Add : Sum  Inputs=+-
  Add1 : Sum
  Add2 : Sum
  Product : Product
  Product1 : Product
  phi1_hat_dot : Outport
  wires:
  eta/1 -> Product/2
  l1/1 -> Product/1
  phi1_hat/1 -> Add/2
  y/1 -> Add/1
  Product/1 -> Product1/1
  Add/1 -> Product1/2
  Product1/1 -> Add1/2
  d1_hat/1 -> Add1/1
  Add1/1 -> Add2/2
  phi2_hat/1 -> Add2/1
  Add2/1 -> phi1_hat_dot/1

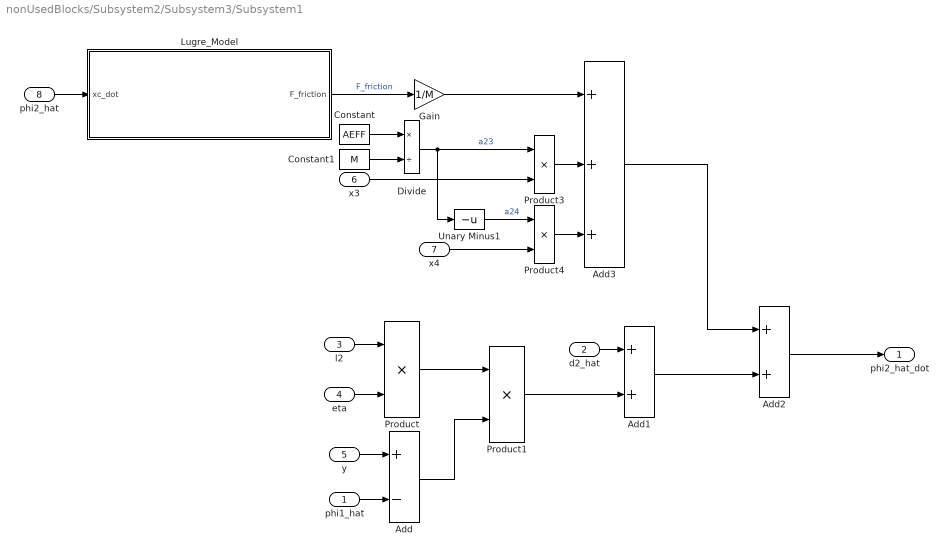
== system nonUsedBlocks/Subsystem2/Subsystem3/Subsystem1 ==
  phi1_hat : Inport
  d2_hat : Inport  Port=2
  l2 : Inport  Port=3
  eta : Inport  Port=4
  y : Inport  Port=5
  x3 : Inport  Port=6
  x4 : Inport  Port=7
  phi2_hat : Inport  Port=8
  Add : Sum  Inputs=+-
  Add1 : Sum
  Add2 : Sum
  Add3 : Sum  Inputs=+++
  Constant : Constant  Value=AEFF
  Constant1 : Constant  Value=M
  Divide : Product  Inputs=*/  RndMeth=Zero  SaturateOnIntegerOverflow=on
  Gain : Gain  Gain=1/M
  Lugre_Model : Subsystem
  Product{,1,3..4} (4 alike) : Product
  Unary Minus1 : UnaryMinus
  phi2_hat_dot : Outport
  wires:
  Add2/1 -> phi2_hat_dot/1
  Add1/1 -> Add2/2
  d2_hat/1 -> Add1/1
  Product1/1 -> Add1/2
  Add/1 -> Product1/2
  Product/1 -> Product1/1
  y/1 -> Add/1
  phi1_hat/1 -> Add/2
  l2/1 -> Product/1
  eta/1 -> Product/2
  Divide/1 -> Product3/1, Unary Minus1/1  "a23"
  x3/1 -> Product3/2
  Unary Minus1/1 -> Product4/1  "a24"
  x4/1 -> Product4/2
  Product3/1 -> Add3/2
  Product4/1 -> Add3/3
  Add3/1 -> Add2/1
  phi2_hat/1 -> Lugre_Model/1(xc_dot)
  Gain/1 -> Add3/1
  Lugre_Model/1(F_friction) -> Gain/1  "F_friction"
  Constant/1 -> Divide/1
  Constant1/1 -> Divide/2

== system nonUsedBlocks/Subsystem2/Subsystem3/Subsystem3 ==
  phi2_hat : Inport
  gamma1 : Inport  Port=2
  phi1_hat : Inport  Port=3
  sigma1_hat : Inport  Port=4
  Add : Sum
  Add1 : Sum
  Product : Product
  Product1 : Product
  Unary Minus : UnaryMinus
  sigma1_hat_dot : Outport
  wires:
  sigma1_hat/1 -> Add/1
  Product/1 -> Add/2
  Add/1 -> Add1/2
  phi2_hat/1 -> Add1/1
  gamma1/1 -> Unary Minus/1, Product/2
  phi1_hat/1 -> Product/1
  Add1/1 -> Product1/1
  Unary Minus/1 -> Product1/2
  Product1/1 -> sigma1_hat_dot/1

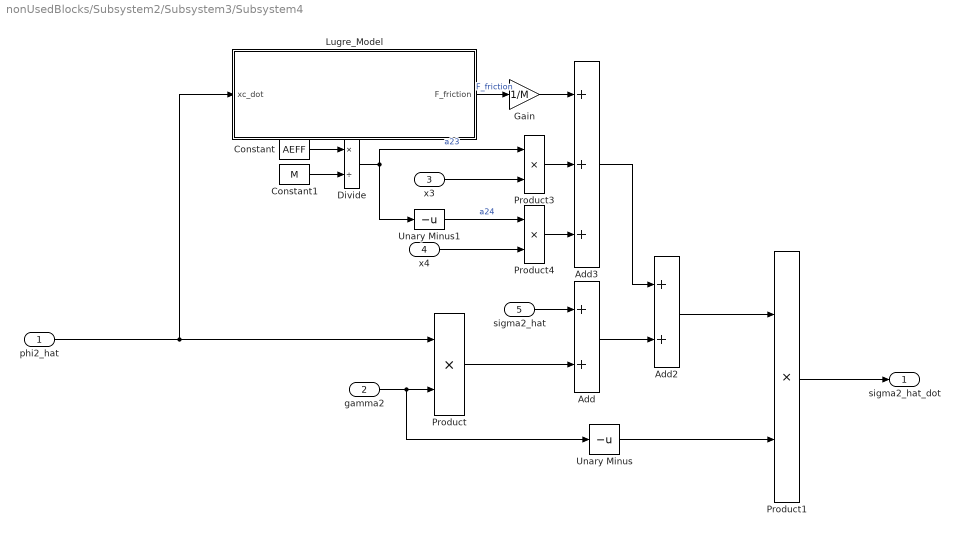
== system nonUsedBlocks/Subsystem2/Subsystem3/Subsystem4 ==
  phi2_hat : Inport
  gamma2 : Inport  Port=2
  x3 : Inport  Port=3
  x4 : Inport  Port=4
  sigma2_hat : Inport  Port=5
  Add : Sum
  Add2 : Sum
  Add3 : Sum  Inputs=+++
  Constant : Constant  Value=AEFF
  Constant1 : Constant  Value=M
  Divide : Product  Inputs=*/  RndMeth=Zero  SaturateOnIntegerOverflow=on
  Gain : Gain  Gain=1/M
  Lugre_Model : Subsystem
  Product{,1,3..4} (4 alike) : Product
  Unary Minus : UnaryMinus
  Unary Minus1 : UnaryMinus
  sigma2_hat_dot : Outport
  wires:
  Product1/1 -> sigma2_hat_dot/1
  gamma2/1 -> Unary Minus/1, Product/2
  Product/1 -> Add/2
  sigma2_hat/1 -> Add/1
  Product3/1 -> Add3/2
  Product4/1 -> Add3/3
  x4/1 -> Product4/2
  phi2_hat/1 -> Product/1, Lugre_Model/1(xc_dot)
  Unary Minus1/1 -> Product4/1  "a24"
  x3/1 -> Product3/2
  Add3/1 -> Add2/1
  Gain/1 -> Add3/1
  Add/1 -> Add2/2
  Add2/1 -> Product1/1
  Unary Minus/1 -> Product1/2
  Lugre_Model/1(F_friction) -> Gain/1  "F_friction"
  Constant/1 -> Divide/1
  Divide/1 -> Product3/1, Unary Minus1/1  "a23"
  Constant1/1 -> Divide/2

== system nonUsedBlocks/Subsystem2/Subsystem3/Subsystem6 ==
  sigma1_hat : Inport
  gamma1 : Inport  Port=2
  phi1_hat : Inport  Port=3
  Add : Sum
  Product : Product
  d1_hat : Outport
  wires:
  sigma1_hat/1 -> Add/1
  gamma1/1 -> Product/1
  phi1_hat/1 -> Product/2
  Product/1 -> Add/2
  Add/1 -> d1_hat/1

== system nonUsedBlocks/Subsystem2/Subsystem3/Subsystem7 ==
  sigma2_hat : Inport
  gamma2 : Inport  Port=2
  phi2_hat : Inport  Port=3
  Add : Sum
  Product : Product
  d2_hat : Outport
  wires:
  gamma2/1 -> Product/1
  sigma2_hat/1 -> Add/1
  Product/1 -> Add/2
  Add/1 -> d2_hat/1
  phi2_hat/1 -> Product/2

== system nonUsedBlocks/old/Flow_Calc_NoLeak/Subsystem1 ==
  Constant : Constant  Value=Cd_pos
  Constant1 : Constant  Value=W
  Constant2 : Constant  Value=RHO
  Constant3 : Constant  Value=2
  Math Reciprocal : Math  Operator=reciprocal  SignedPower=on
  Product : Product  Inputs=3
  Product1 : Product
  Sqrt : Sqrt
  Kq : Outport
  wires:
  Product/1 -> Kq/1
  Sqrt/1 -> Product/3
  Product1/1 -> Sqrt/1
  Constant3/1 -> Product1/1
  Math Reciprocal/1 -> Product1/2
  Constant2/1 -> Math Reciprocal/1  "rho"
  Constant1/1 -> Product/2  "w"
  Constant/1 -> Product/1  "Cd"

== system nonUsedBlocks/old/Flow_Calc_NoLeak/Subsystem2 ==
  Constant : Constant  Value=Cd_neg
  Constant1 : Constant  Value=W
  Constant2 : Constant  Value=RHO
  Constant3 : Constant  Value=2
  Math Reciprocal : Math  Operator=reciprocal  SignedPower=on
  Product : Product  Inputs=3
  Product1 : Product
  Sqrt : Sqrt
  Kq : Outport
  wires:
  Constant/1 -> Product/1  "Cd"
  Constant1/1 -> Product/2  "w"
  Constant2/1 -> Math Reciprocal/1  "rho"
  Math Reciprocal/1 -> Product1/2
  Constant3/1 -> Product1/1
  Product1/1 -> Sqrt/1
  Sqrt/1 -> Product/3
  Product/1 -> Kq/1

== system nonUsedBlocks/old/ServoValve_Dynamics/Convert_SpoolPosition ==
  u_perc : Inport  OutDataTypeStr=double
  Constant : Constant  Value=50e-3
  Constant1 : Constant  Value=0.01
  Constant2 : Constant  Value=0.001016
  Constant3 : Constant  Value=50e-3
  Math Reciprocal : Math  Operator=reciprocal  SignedPower=on
  Product : Product  Inputs=3
  Product1 : Product
  Product2 : Product
  xv : Outport  OutDataTypeStr=double
  wires:
  u_perc/1 -> Product/3
  Constant1/1 -> Product/2
  Constant3/1 -> Product/1
  Constant2/1 -> Product1/1
  Math Reciprocal/1 -> Product1/2
  Constant/1 -> Math Reciprocal/1
  Product1/1 -> Product2/2  "Ki"
  Product/1 -> Product2/1  "i"
  Product2/1 -> xv/1  "xv"

== system nonUsedBlocks/old/ServoValve_Dynamics/Subsystem ==
  Valve Dynamics1 : TransferFcn  Numerator=[7.738e05]  Denominator=[1 1244 7.738e05]
  Valve Dynamics2 : TransferFcn  Numerator=[(120*2*pi)^2]  Denominator=[1 2*0.95*(120*2*pi) (120*2*pi)^2]

== system nonUsedBlocks/Nguyen Observer/Nguyen_Observer/phi_calc/Delta_1 ==
  x1 : Inport
  Add2 : Sum
  Constant5 : Constant  Value=B_E
  Constant6 : Constant  Value=AEFF
  Constant7 : Constant  Value=V01
  Gain : Gain  Gain=1e-2
  Math Reciprocal : Math  Operator=reciprocal  SignedPower=on
  Product5 : Product
  Product6 : Product
  Delta_1 : Outport
  wires:
  Product5/1 -> Add2/2
  Constant5/1 -> Gain/1
  Math Reciprocal/1 -> Product6/2
  x1/1 -> Product5/2
  Product6/1 -> Delta_1/1
  Add2/1 -> Math Reciprocal/1
  Constant6/1 -> Product5/1
  Constant7/1 -> Add2/1
  Gain/1 -> Product6/1

== system nonUsedBlocks/Nguyen Observer/Nguyen_Observer/phi_calc/Delta_2 ==
  x1 : Inport
  Add2 : Sum  Inputs=+-
  Constant5 : Constant  Value=B_E
  Constant6 : Constant  Value=AEFF
  Constant7 : Constant  Value=V02
  Gain2 : Gain  Gain=1e-2
  Math Reciprocal : Math  Operator=reciprocal  SignedPower=on
  Product5 : Product
  Product6 : Product
  Delta_2 : Outport
  wires:
  Add2/1 -> Math Reciprocal/1
  Product6/1 -> Delta_2/1
  x1/1 -> Product5/2
  Math Reciprocal/1 -> Product6/2
  Constant5/1 -> Gain2/1
  Product5/1 -> Add2/2
  Constant6/1 -> Product5/1
  Constant7/1 -> Add2/1
  Gain2/1 -> Product6/1

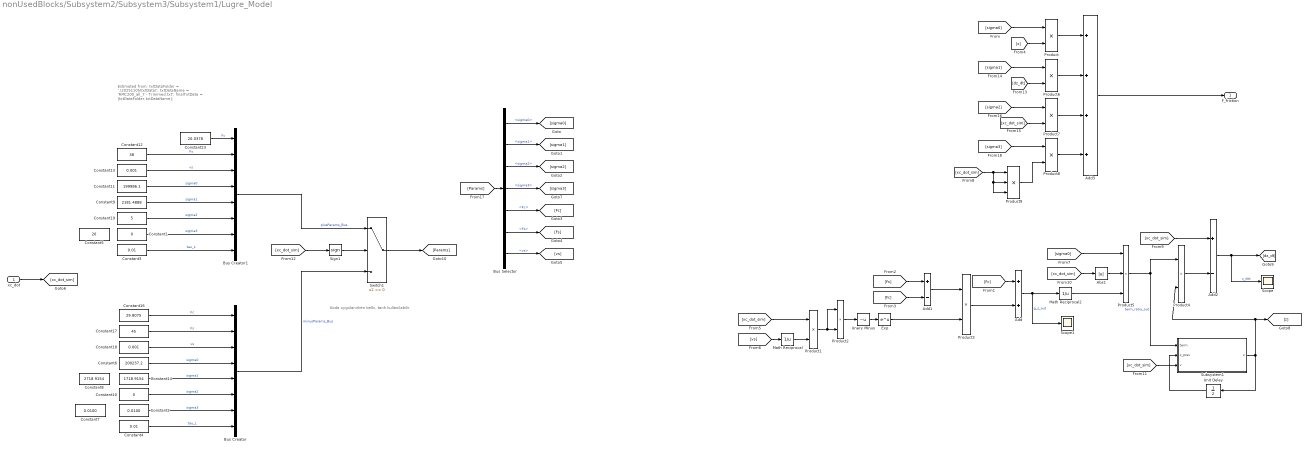
== system nonUsedBlocks/Subsystem2/Subsystem3/Subsystem1/Lugre_Model ==
  note: Koda uygulanırken belki, tanh kullanılabilir
  note: Estimated from:
      |
      | txtDataFolder = '.\20251105\txtData\';
      | txtDataName = 'RMC200_all_7 - Trimmed.txt';
      | finalTxtData = [txtDataFolder,txtDataName];
  xc_dot : Inport  OutDataTypeStr=double
  Abs1 : Abs  SaturateOnIntegerOverflow=off
  Add : Sum
  Add1 : Sum  Inputs=+-
  Add2 : Sum  Inputs=+-
  Add3 : Sum  Inputs=++++
  Bus Selector : BusSelector  OutputSignals=sigma0,sigma1,sigma2,sigma3,Fc,Fs,vs
  Bus Creator : BusCreator  Inputs=8
  Bus Creator1 : BusCreator  Inputs=8
  Constant1 : Constant  Value=0  OutDataTypeStr=double
  Constant10 : Constant  Value=0  OutDataTypeStr=double
  Constant11 : Constant  Value=199986.1  OutDataTypeStr=double
  Constant12 : Constant  Value=38  OutDataTypeStr=double
  Constant13 : Constant  Value=0.001  OutDataTypeStr=double
  Constant14 : Constant  Value=1718.9154  OutDataTypeStr=double
  Constant16 : Constant  Value=29.8075  OutDataTypeStr=double
  Constant17 : Constant  Value=45  OutDataTypeStr=double
  Constant18 : Constant  Value=0.001  OutDataTypeStr=double
  Constant19 : Constant  Value=5  OutDataTypeStr=double
  Constant2 : Constant  Value=0.0100  OutDataTypeStr=double
  Constant23 : Constant  Value=20.0378  OutDataTypeStr=double
  Constant3 : Constant  Value=0.01  OutDataTypeStr=double
  Constant4 : Constant  Value=0.01  OutDataTypeStr=double
  Constant5 : Constant  Value=20  OutDataTypeStr=double
  Constant6 : Constant  Value=200237.2  OutDataTypeStr=double
  Constant7 : Constant  Value=0.0100  OutDataTypeStr=double
  Constant8 : Constant  Value=2718.9154  OutDataTypeStr=double
  Constant9 : Constant  Value=2181.4888  OutDataTypeStr=double
  Exp : Math  SignedPower=on
  Math Reciprocal : Math  Operator=reciprocal  SignedPower=on
  Math Reciprocal2 : Math  Operator=reciprocal  SignedPower=on
  Product{,1..4,6..8} (8 alike) : Product
  Product5 : Product  Inputs=3
  Product9 : Product  Inputs=3
  Scope : Scope
  Scope1 : Scope
  Sign1 : Signum
  Subsystem1 : Subsystem
  Switch1 : Switch  SaturateOnIntegerOverflow=off  InputSameDT=off
  Unary Minus : UnaryMinus
  Unit Delay : UnitDelay  SampleTime=-1  HasFrameUpgradeWarning=on
  F_friction : Outport
  wires:
  Constant18/1 -> Bus Creator/3  "vs"
  Constant13/1 -> Bus Creator1/3  "vs"
  Constant12/1 -> Bus Creator1/2  "Fs"
  Constant17/1 -> Bus Creator/2  "Fs"
  Constant14/1 -> Bus Creator/5  "sigma1"
  Constant6/1 -> Bus Creator/4  "sigma0"
  Constant10/1 -> Bus Creator/6  "sigma2"
  Constant16/1 -> Bus Creator/1  "Fc"
  Constant9/1 -> Bus Creator1/5  "sigma1"
  Constant11/1 -> Bus Creator1/4  "sigma0"
  Constant19/1 -> Bus Creator1/6  "sigma2"
  Product7/1 -> Add3/3
  Product6/1 -> Add3/2
  [sigma2] -> Product7/1
  [xc_dot_sim] -> Product7/2
  [dz_dt] -> Product6/2
  [sigma1] -> Product6/1
  Product/1 -> Add3/1
  [z] -> Product/2
  [sigma0] -> Product5/1
  Abs1/1 -> Product5/2
  Add/1 -> Math Reciprocal2/1, Scope1/1  "g_s_out"
  [xc_dot_sim] -> Abs1/1
  Add1/1 -> Product3/1
  Unary Minus/1 -> Exp/1
  Product2/1 -> Unary Minus/1
  Product1/1 -> Product2/2, Product2/1
  [xc_dot_sim] -> Product1/1
  Math Reciprocal/1 -> Product1/2
  [vs] -> Math Reciprocal/1
  [Fc] -> Add1/2
  [Fs] -> Add1/1
  [Fc] -> Add/1
  [sigma0] -> Product/1
  Product3/1 -> Add/2
  [xc_dot_sim] -> Sign1/1
  Bus Creator1/1 -> Switch1/1  "plusParams_Bus"
  Bus Creator/1 -> Switch1/3  "minusParams_Bus"
  Switch1/1 -> [Params]
  [Params] -> Bus Selector/1
  Bus Selector/1 -> [sigma0]  "<sigma0>"
  Bus Selector/2 -> [sigma1]  "<sigma1>"
  Bus Selector/3 -> [sigma2]  "<sigma2>"
  Bus Selector/5 -> [Fc]  "<Fc>"
  Bus Selector/6 -> [Fs]  "<Fs>"
  Bus Selector/7 -> [vs]  "<vs>"
  Math Reciprocal2/1 -> Product5/3
  Exp/1 -> Product3/2
  Add2/1 -> Scope/1, [dz_dt]  "z_dot"
  Sign1/1 -> Switch1/2
  [xc_dot_sim] -> Add2/1
  Subsystem1/1(z) -> Product4/2, [z], Unit Delay/1
  [xc_dot_sim] -> Subsystem1/3(v)
  Unit Delay/1 -> Subsystem1/2(z_prev)
  Product5/1 -> Subsystem1/1(term), Product4/1  "term_ratio_out"
  Product4/1 -> Add2/2
  Add3/1 -> F_friction/1
  Constant1/1 -> Bus Creator1/7  "sigma3"
  Constant2/1 -> Bus Creator/7  "sigma3"
  Constant3/1 -> Bus Creator1/8  "tau_L"
  Constant4/1 -> Bus Creator/8  "tau_L"
  [sigma3] -> Product8/1
  Product8/1 -> Add3/4
  [xc_dot_sim] -> Product9/2, Product9/3, Product9/1
  Product9/1 -> Product8/2
  Bus Selector/4 -> [sigma3]  "<sigma3>"
  xc_dot/1 -> [xc_dot_sim]
  Constant23/1 -> Bus Creator1/1  "Fc"

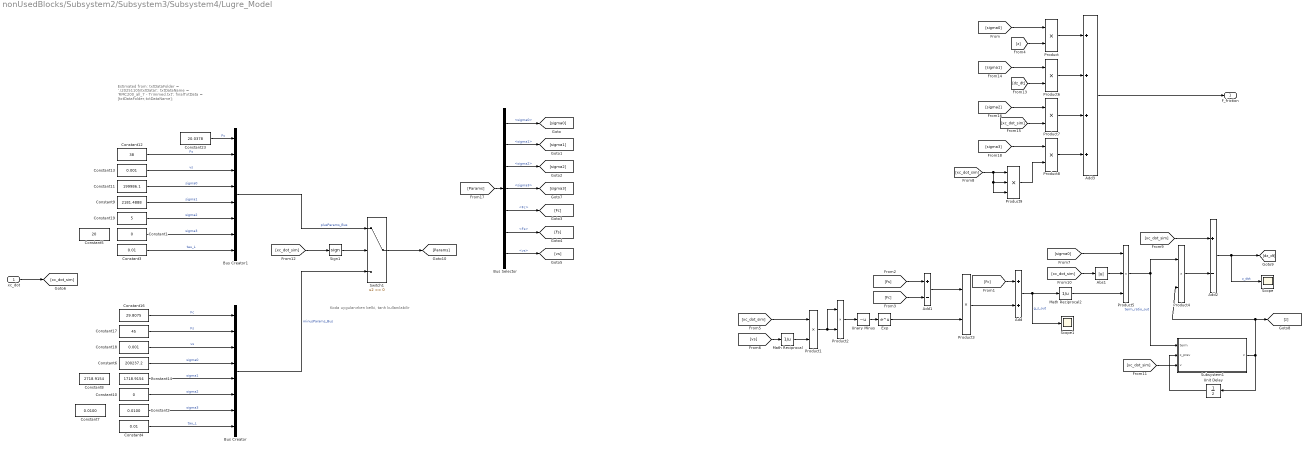
== system nonUsedBlocks/Subsystem2/Subsystem3/Subsystem4/Lugre_Model ==
  note: Koda uygulanırken belki, tanh kullanılabilir
  note: Estimated from:
      |
      | txtDataFolder = '.\20251105\txtData\';
      | txtDataName = 'RMC200_all_7 - Trimmed.txt';
      | finalTxtData = [txtDataFolder,txtDataName];
  xc_dot : Inport  OutDataTypeStr=double
  Abs1 : Abs  SaturateOnIntegerOverflow=off
  Add : Sum
  Add1 : Sum  Inputs=+-
  Add2 : Sum  Inputs=+-
  Add3 : Sum  Inputs=++++
  Bus Selector : BusSelector  OutputSignals=sigma0,sigma1,sigma2,sigma3,Fc,Fs,vs
  Bus Creator : BusCreator  Inputs=8
  Bus Creator1 : BusCreator  Inputs=8
  Constant1 : Constant  Value=0  OutDataTypeStr=double
  Constant10 : Constant  Value=0  OutDataTypeStr=double
  Constant11 : Constant  Value=199986.1  OutDataTypeStr=double
  Constant12 : Constant  Value=38  OutDataTypeStr=double
  Constant13 : Constant  Value=0.001  OutDataTypeStr=double
  Constant14 : Constant  Value=1718.9154  OutDataTypeStr=double
  Constant16 : Constant  Value=29.8075  OutDataTypeStr=double
  Constant17 : Constant  Value=45  OutDataTypeStr=double
  Constant18 : Constant  Value=0.001  OutDataTypeStr=double
  Constant19 : Constant  Value=5  OutDataTypeStr=double
  Constant2 : Constant  Value=0.0100  OutDataTypeStr=double
  Constant23 : Constant  Value=20.0378  OutDataTypeStr=double
  Constant3 : Constant  Value=0.01  OutDataTypeStr=double
  Constant4 : Constant  Value=0.01  OutDataTypeStr=double
  Constant5 : Constant  Value=20  OutDataTypeStr=double
  Constant6 : Constant  Value=200237.2  OutDataTypeStr=double
  Constant7 : Constant  Value=0.0100  OutDataTypeStr=double
  Constant8 : Constant  Value=2718.9154  OutDataTypeStr=double
  Constant9 : Constant  Value=2181.4888  OutDataTypeStr=double
  Exp : Math  SignedPower=on
  Math Reciprocal : Math  Operator=reciprocal  SignedPower=on
  Math Reciprocal2 : Math  Operator=reciprocal  SignedPower=on
  Product{,1..4,6..8} (8 alike) : Product
  Product5 : Product  Inputs=3
  Product9 : Product  Inputs=3
  Scope : Scope
  Scope1 : Scope
  Sign1 : Signum
  Subsystem1 : Subsystem
  Switch1 : Switch  SaturateOnIntegerOverflow=off  InputSameDT=off
  Unary Minus : UnaryMinus
  Unit Delay : UnitDelay  SampleTime=-1  HasFrameUpgradeWarning=on
  F_friction : Outport
  wires:
  Constant18/1 -> Bus Creator/3  "vs"
  Constant13/1 -> Bus Creator1/3  "vs"
  Constant12/1 -> Bus Creator1/2  "Fs"
  Constant17/1 -> Bus Creator/2  "Fs"
  Constant14/1 -> Bus Creator/5  "sigma1"
  Constant6/1 -> Bus Creator/4  "sigma0"
  Constant10/1 -> Bus Creator/6  "sigma2"
  Constant16/1 -> Bus Creator/1  "Fc"
  Constant9/1 -> Bus Creator1/5  "sigma1"
  Constant11/1 -> Bus Creator1/4  "sigma0"
  Constant19/1 -> Bus Creator1/6  "sigma2"
  Product7/1 -> Add3/3
  Product6/1 -> Add3/2
  [sigma2] -> Product7/1
  [xc_dot_sim] -> Product7/2
  [dz_dt] -> Product6/2
  [sigma1] -> Product6/1
  Product/1 -> Add3/1
  [z] -> Product/2
  [sigma0] -> Product5/1
  Abs1/1 -> Product5/2
  Add/1 -> Math Reciprocal2/1, Scope1/1  "g_s_out"
  [xc_dot_sim] -> Abs1/1
  Add1/1 -> Product3/1
  Unary Minus/1 -> Exp/1
  Product2/1 -> Unary Minus/1
  Product1/1 -> Product2/2, Product2/1
  [xc_dot_sim] -> Product1/1
  Math Reciprocal/1 -> Product1/2
  [vs] -> Math Reciprocal/1
  [Fc] -> Add1/2
  [Fs] -> Add1/1
  [Fc] -> Add/1
  [sigma0] -> Product/1
  Product3/1 -> Add/2
  [xc_dot_sim] -> Sign1/1
  Bus Creator1/1 -> Switch1/1  "plusParams_Bus"
  Bus Creator/1 -> Switch1/3  "minusParams_Bus"
  Switch1/1 -> [Params]
  [Params] -> Bus Selector/1
  Bus Selector/1 -> [sigma0]  "<sigma0>"
  Bus Selector/2 -> [sigma1]  "<sigma1>"
  Bus Selector/3 -> [sigma2]  "<sigma2>"
  Bus Selector/5 -> [Fc]  "<Fc>"
  Bus Selector/6 -> [Fs]  "<Fs>"
  Bus Selector/7 -> [vs]  "<vs>"
  Math Reciprocal2/1 -> Product5/3
  Exp/1 -> Product3/2
  Add2/1 -> Scope/1, [dz_dt]  "z_dot"
  Sign1/1 -> Switch1/2
  [xc_dot_sim] -> Add2/1
  Subsystem1/1(z) -> Product4/2, [z], Unit Delay/1
  [xc_dot_sim] -> Subsystem1/3(v)
  Unit Delay/1 -> Subsystem1/2(z_prev)
  Product5/1 -> Subsystem1/1(term), Product4/1  "term_ratio_out"
  Product4/1 -> Add2/2
  Add3/1 -> F_friction/1
  Constant1/1 -> Bus Creator1/7  "sigma3"
  Constant2/1 -> Bus Creator/7  "sigma3"
  Constant3/1 -> Bus Creator1/8  "tau_L"
  Constant4/1 -> Bus Creator/8  "tau_L"
  [sigma3] -> Product8/1
  Product8/1 -> Add3/4
  [xc_dot_sim] -> Product9/2, Product9/3, Product9/1
  Product9/1 -> Product8/2
  Bus Selector/4 -> [sigma3]  "<sigma3>"
  xc_dot/1 -> [xc_dot_sim]
  Constant23/1 -> Bus Creator1/1  "Fc"

== system nonUsedBlocks/Subsystem2/Subsystem3/Subsystem1/Lugre_Model/Subsystem1 ==
  term : Inport
  z_prev : Inport  Port=2
  v : Inport  Port=3
  Add : Sum
  Add1 : Sum
  Constant : Constant
  Gain : Gain  Gain=1e-3
  Gain1 : Gain  Gain=1e-3
  Math Reciprocal2 : Math  Operator=reciprocal  SignedPower=on
  Product : Product
  z : Outport
  wires:
  term/1 -> Gain1/1
  z_prev/1 -> Add/1
  v/1 -> Gain/1
  Gain/1 -> Add/2
  Add/1 -> Product/1
  Gain1/1 -> Add1/2
  Constant/1 -> Add1/1
  Add1/1 -> Math Reciprocal2/1
  Math Reciprocal2/1 -> Product/2
  Product/1 -> z/1

== system nonUsedBlocks/Subsystem2/Subsystem3/Subsystem4/Lugre_Model/Subsystem1 ==
  term : Inport
  z_prev : Inport  Port=2
  v : Inport  Port=3
  Add : Sum
  Add1 : Sum
  Constant : Constant
  Gain : Gain  Gain=1e-3
  Gain1 : Gain  Gain=1e-3
  Math Reciprocal2 : Math  Operator=reciprocal  SignedPower=on
  Product : Product
  z : Outport
  wires:
  term/1 -> Gain1/1
  z_prev/1 -> Add/1
  v/1 -> Gain/1
  Gain/1 -> Add/2
  Add/1 -> Product/1
  Gain1/1 -> Add1/2
  Constant/1 -> Add1/1
  Add1/1 -> Math Reciprocal2/1
  Math Reciprocal2/1 -> Product/2
  Product/1 -> z/1

== matlab function nonUsedBlocks/old/MATLAB Function2 ==
  data: xv input; Q1 output; P_P input; P_T input; P_A input; P_B input; Q2 output; Q_RETURN output
function [Q1, Q2, Q_RETURN] = fcn_Valve_Tamburrano_Hybrid( ...
    xv, P_P, P_T, P_A, P_B)

% SI units:
% xv [m], P_* [Pa], w,c,r [m], rho [kg/m^3], mu [Pa*s], Cd [-]
%
% Outputs:
%   Q_A, Q_B         : Port net flows [m^3/s]
%   Q_Leak_Total     : leakage indicator [m^3/s]
%   Q_return_lpm     : total return flow to return line [LPM]

%% 0) Checks

%%
k = 0.2; 
K = 1.7817e-6; 
x0 = 0.00099959586;

x = xv;
P_S = P_P;
P_A = P_A; 
P_B = P_B;
P_R = P_T;

K1_S = K;
K1_R = K; 
K2_S = K; 
K2_R = K; 

k1_s = k; 
k1_r = k; 
k2_s = k; 
k2_r = k; 

%% 
if x >= 0
        % For control port 1
        Q1_S = K1_S * sqrt(abs(P_S - P_A)) * (x0 + x) * sign(P_S - P_A);
        Q1_R = K1_R * sqrt(abs(P_A - P_R)) * (x0^2) * ((x0 + k1_r*x)^-1) *sign(P_A - P_R);

        % For control port 2
        Q2_S = K2_S * sqrt(abs(P_S - P_B)) * (x0^2) * ((x0 + k2_s*x)^-1) *sign((P_S - P_B)); 
        Q2_R = K2_R * sqrt(abs(P_B - P_R)) * (x0 + x) * sign((P_B - P_R)); 
else 
        % For control port 1
        Q1_S = K1_S * sqrt(abs(P_S - P_A)) * (x0^2) * ((x0 - k1_s*x)^-1) * sign(P_S - P_A);
        Q1_R = K1_R * sqrt(abs(P_A - P_R)) * (x0 - x) * sign(P_A - P_R);

        % For control port 2
        Q2_S = K2_S * sqrt(abs(P_S - P_B)) * (x0 - x) * sign(P_S - P_B); 
        Q2_R = K2_R * sqrt(abs(P_B - P_R)) * (x0^2) * ((x0 - k2_r*x)^-1)* sign(P_B - P_R); 
end 

Q1 = Q1_S - Q1_R; 
Q2 = Q2_S - Q2_R; 

Q_RETURN = Q1_R + Q2_R;
